simulink model "Process_IMU_Data"  (R2016a)
settings: Solver=VariableStepAuto  StartTime=0.0  StopTime=10.0  RelTol=1e-3
undefined symbols (not defined in the file or in its folder): DiscIntNeverNeededParam
settings Model: Creator=sannem  LastModifiedBy=sannem
settings RTWCC: GenerateReport=on  LaunchReport=on
settings GRTTargetCC: GeneratePreprocessorConditionals=Use local settings

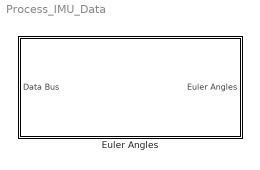
== system Process_IMU_Data ==
  Euler Angles : Subsystem

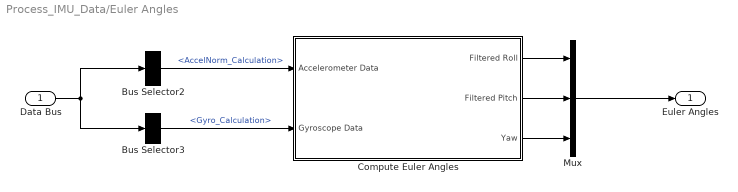
== system Process_IMU_Data/Euler Angles ==
  Data Bus : Inport  OutDataTypeStr=Bus: Measurement_Calculation_Bus
  Bus Selector2 : BusSelector  OutputSignals=AccelNorm_Calculation
  Bus Selector3 : BusSelector  OutputSignals=Gyro_Calculation
  Compute Euler Angles : Subsystem
  Mux : Mux  Inputs=3
  Euler Angles : Outport
  wires:
  Data Bus/1 -> Bus Selector3/1, Bus Selector2/1
  Bus Selector3/1 -> Compute Euler Angles/2(Gyroscope Data)  "<Gyro_Calculation>"
  Bus Selector2/1 -> Compute Euler Angles/1(Accelerometer Data)  "<AccelNorm_Calculation>"
  Mux/1 -> Euler Angles/1
  Compute Euler Angles/1(Filtered Roll) -> Mux/1
  Compute Euler Angles/2(Filtered Pitch) -> Mux/2
  Compute Euler Angles/3(Yaw) -> Mux/3

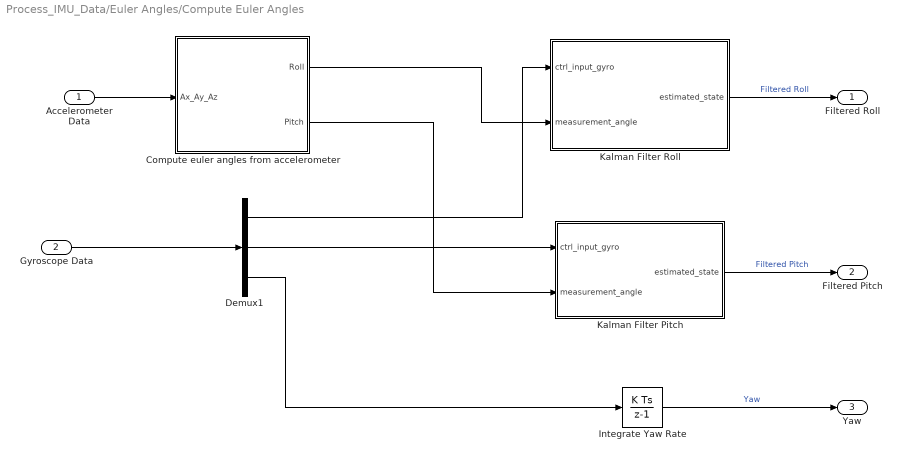
== system Process_IMU_Data/Euler Angles/Compute Euler Angles ==
  Accelerometer Data : Inport
  Gyroscope Data : Inport  Port=2
  Compute euler angles from accelerometer : MATLAB Function  TreatAsAtomicUnit=on
  Demux1 : Demux  Outputs=3
  Integrate Yaw Rate : DiscreteIntegrator  SampleTime=1/400  OutDataTypeStr=double  ICPrevOutput=DiscIntNeverNeededParam  ICPrevScaledInput=DiscIntNeverNeededParam
  Kalman Filter Pitch : MATLAB Function  TreatAsAtomicUnit=on
  Kalman Filter Roll : MATLAB Function  TreatAsAtomicUnit=on
  Filtered Roll : Outport
  Filtered Pitch : Outport  Port=2
  Yaw : Outport  Port=3
  wires:
  Compute euler angles from accelerometer/2(Pitch) -> Kalman Filter Pitch/2(measurement_angle)
  Integrate Yaw Rate/1 -> Yaw/1  "Yaw"
  Kalman Filter Roll/1(estimated_state) -> Filtered Roll/1  "Filtered Roll"
  Demux1/3 -> Integrate Yaw Rate/1
  Demux1/2 -> Kalman Filter Pitch/1(ctrl_input_gyro)
  Kalman Filter Pitch/1(estimated_state) -> Filtered Pitch/1  "Filtered Pitch"
  Demux1/1 -> Kalman Filter Roll/1(ctrl_input_gyro)
  Compute euler angles from accelerometer/1(Roll) -> Kalman Filter Roll/2(measurement_angle)
  Accelerometer Data/1 -> Compute euler angles from accelerometer/1(Ax_Ay_Az)
  Gyroscope Data/1 -> Demux1/1

== matlab function Process_IMU_Data/Euler Angles/Compute Euler Angles/Compute euler angles from accelerometer ==
  data: Ax_Ay_Az input; Roll output; Pitch output
function [Roll,Pitch] = CalculateAngle(Ax_Ay_Az)

% using the method as described in
% http://www.digikey.com/en/articles/techzone/2011/may/using-an-accelerometer-for-inclination-sensing
%#codegen
Ax = -Ax_Ay_Az(1);
Ay = -Ax_Ay_Az(2);
Az = Ax_Ay_Az(3);

Roll = 180 / pi * atan( Ay / sqrt( Ax^2 + Az^2));
Pitch = -180 / pi * atan( Ax / sqrt( Ay^2 + Az^2));

== matlab function Process_IMU_Data/Euler Angles/Compute Euler Angles/Kalman Filter Roll ==
  data: estimated_state output; ctrl_input_gyro input; measurement_angle input
function estimated_state  = fcn( ctrl_input_gyro, measurement_angle)

persistent prev_state
if isempty(prev_state)
    prev_state = [0;0];
end
persistent covariance_correction_prev
if isempty(covariance_correction_prev)
    covariance_correction_prev = eye(2);
end

%-------------------------------
%-------------------------------
%---- Predict Stage ------------
%-------------------------------
%-------------------------------
% pix_value = 5;
Ts = 1/400;
%Process Noise
p_var =0.01;
Q = [p_var^2     0         
      0         p_var^2];

%A matrix
A =  [1   -Ts 
      0   1];

%odutput these values with a unit delay (for algebraic loop), apply initial conditions
state_prediction = A*prev_state + [Ts 0; 0 0]*[ctrl_input_gyro; 0 ];
covariance_prediction = A*covariance_correction_prev*A' + Q;

%-------------------------------
%-------------------------------
%---- Estimate Stage -----------
%-------------------------------
%-------------------------------

%H matrix
H = [1 0];

%Measurement noise from accelerometer angle measurement
m_var = 0.5;
R = [m_var^2 ];

%Measurement Z
Z = [measurement_angle];

%Compute Kalman Gain
Kalman_Gain = covariance_prediction*H'*inv(H*covariance_prediction*H'+R); %2x2 matrix

%compute state space correction based on measurement
state_correction = state_prediction + Kalman_Gain*(Z - H*state_prediction); %4x1 vector of states

%compute covariance correction
covariance_correction = (eye(2) - Kalman_Gain*H)*covariance_prediction; %2x2 covariance matrix

%save the found values for the next sample
estimated_state = state_correction (1);
prev_state = state_correction;
covariance_correction_prev = covariance_correction;
 end

== matlab function Process_IMU_Data/Euler Angles/Compute Euler Angles/Kalman Filter Pitch ==
  data: estimated_state output; ctrl_input_gyro input; measurement_angle input
function estimated_state  = fcn(ctrl_input_gyro, measurement_angle)


persistent prev_state
if isempty(prev_state)
    prev_state = [0;0];
end
persistent covariance_correction_prev
if isempty(covariance_correction_prev)
    covariance_correction_prev = eye(2);
end


%-------------------------------
%-------------------------------
%---- Predict Stage ------------
%-------------------------------
%-------------------------------
% pix_value = 5;
Ts = 1/400;
%Process Noise
p_var =0.01;
Q = [p_var^2     0         
      0         p_var^2];

%A matrix
A =  [1   -Ts 
      0   1];

%odutput these values with a unit delay (for algebraic loop), apply initial conditions
state_prediction = A*prev_state + [Ts 0; 0 0]*[ctrl_input_gyro; 0 ];
covariance_prediction = A*covariance_correction_prev*A' + Q;

%-------------------------------
%-------------------------------
%---- Estimate Stage -----------
%-------------------------------
%-------------------------------

%H matrix
H = [1 0];

%Measurement noise from accelerometer angle measurement
m_var = 1;
%     m_var_r = 1;

R = [m_var^2 ];

%Measurement Z
Z = [measurement_angle];

%Compute Kalman Gain
Kalman_Gain = covariance_prediction*H'*inv(H*covariance_prediction*H'+R); %2x2 matrix

%compute state space correction based on measurement
state_correction = state_prediction + Kalman_Gain*(Z - H*state_prediction); %4x1 vector of states

%compute covariance correction
covariance_correction = (eye(2) - Kalman_Gain*H)*covariance_prediction; %2x2 covariance matrix

%save the found values for the next sample
estimated_state = state_correction (1);
prev_state = state_correction;
covariance_correction_prev = covariance_correction;
end
